simulink model "simscaptestworkspace"  (R2016b)
settings: Solver=VariableStepAuto  StartTime=0.0  StopTime=12100  RelTol=1e-3  AbsTol=1e-3  EnableMultiTasking=on
model workspace (MAT data in the model file):
  OCVdisch = [0  3.706; 5  3.337; 10  3.333; 15  3.331; 20  3.33; 25  3.329; 30  3.3284; 35  3.3272; 40  3.3237; 45  3.309; 50  3.2985; 55  3.295; 60  3.293; 65  3.2914; 70  3.2913; 75  3.2898; 80  3.2878; 85  3.2852; 90  3.2747; 95  3.259; 100  3.249; 105  3.2412; 110  3.231; 115  3.2172; 120  3.1983; 125  3.1673; 130  3.042; 132.5  2.9]
  Var = 1
undefined symbols (not defined in the file): C1, C2, C3, DOD, DOD1, OCV, R0, R1, R2, R3, sigbuilder_block
libraries: nesl_utility x11, fl_lib x8, elec_lib x3
settings Model: Creator=Karel Van Peteghem  LastModifiedBy=Karel Van Peteghem
settings DataIOCC: LimitDataPoints=on
settings OptimizationCC: LifeSpan=inf
settings DebuggingCC: AllowSymbolicDim=off  SFUnexpectedBacktrackingDiag=warning  SFNoUnconditionalDefaultTransitionDiag=warning  SFExecutionAtInitializationDiag=none
settings GRTTargetCC: TargetLangStandard=C89/C90 (ANSI)  GeneratePreprocessorConditionals=Disable all
settings ConfigComp: CovMetricSettings=dw  CovHtmlReporting=on  CovSaveCumulativeToWorkspaceVar=on  CovSaveSingleToWorkspaceVar=on  CovExternalEMLEnable=off  CovSFcnEnable=off
settings SimscapeCC: SimscapeLogType=all  SimscapeLogDataHistory=10000

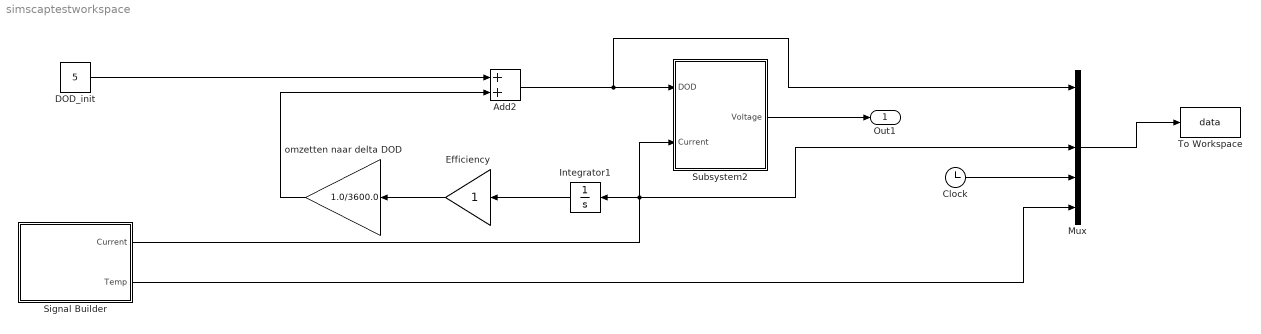
== system simscaptestworkspace ==
  Add2 : Sum
  Clock : Clock
  "DOD_init " : Constant  Value=5
  Efficiency : Gain
  Integrator1 : Integrator
  Mux : Mux  Inputs=5
  Signal Builder : Subsystem  Tag=STV Subsys  LoadFcn=sigbuilder_block('load');  StartFcn=sigbuilder_block('start');  StopFcn=sigbuilder_block('stop');  ClipboardFcn=sigbuilder_block('clipboard');  mask(Sigbuilder block){tuvar=[0:10]}
      mask help: Simulink:masks:SigbuilderBlock_MD
      mask init:
      | if ~strcmp(get_param(bdroot(gcbh),'SimulationStatus'),'stopped') tuvar = sigbuilder_block('maskInit'); end
      settings: CopyFcn=sigbuilder_block('copy');  DeleteFcn=sigbuilder_block('delete');  ModelCloseFcn=sigbuilder_block('modelClose');  PreSaveFcn=sigbuilder_block('preSave');  PauseFcn=sigbuilder_block('pause');  ContinueFcn=sigbuilder_block('continue');  NameChangeFcn=sigbuilder_block('namechange');  OpenFcn=sigbuilder_block('open',[228 111.75 550.5 359.25 ]);  CloseFcn=sigbuilder_block('close');
      mask Display: plot(0, 0, 100, 100,[2, 2, 32, 32, 2], [68, 8, 8, 68, 68],[32, 2], [38, 38], [32, 19, 2],[53, 60, 44], [32, 17, 17, 2],[16, 16, 31, 31]);txt = getActiveGroup(gcbh);text(2, 100, txt,'verticalAlignment', 'top');
  Subsystem2 : Subsystem
  To Workspace : ToWorkspace  VariableName=data  SampleTime=1
  omzetten naar delta DOD : Gain  Gain=1.0/3600.0
  Out1 : Outport
  wires:
  Mux/1 -> To Workspace/1
  "DOD_init "/1 -> Add2/1
  Add2/1 -> Mux/1, Subsystem2/1(DOD)
  Efficiency/1 -> omzetten naar delta DOD/1
  omzetten naar delta DOD/1 -> Add2/2
  Signal Builder/1(Current) -> Mux/3, Integrator1/1, Subsystem2/2(Current)
  Integrator1/1 -> Efficiency/1
  Clock/1 -> Mux/4
  Signal Builder/2(Temp) -> Mux/5
  Subsystem2/1(Voltage) -> Out1/1

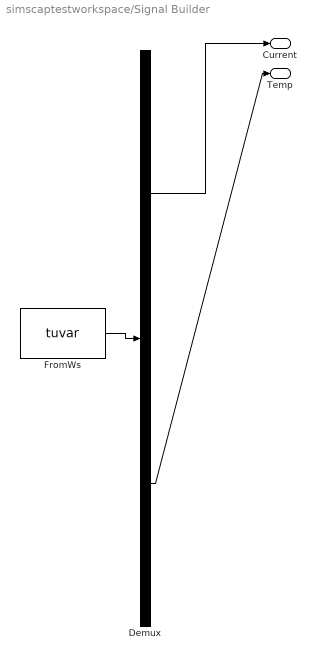
== system simscaptestworkspace/Signal Builder ==
  Demux : Demux  Tag=STV Demux  Outputs=2
  FromWs : FromWorkspace  Tag=STV FromWs  VariableName=tuvar  SampleTime=0
      SigBuilderData=|
      | common.afterFinalStr = 'Extrapolate'
      | common.sampleTime = 0
      | dataSet.timeRange = [0 12000]
      | dataSet.name = 'Blad1'
      | sbobj.Name = 'Signal Builder'
      | sbobj.Groups.Name = 'Blad1'
      | sbobj.Groups.Signals(1).Name = 'Current'
      | sbobj.Groups.Signals(1).XData = [0 101 101 1277 1277 12000]
      | sbobj.Groups.Signals(1).YData = [0 0 15 15 0 0]
      | sbobj.Groups.Signals(2).Name = 'Temp'
      | sbobj.Groups.Signals(2).XData = [0 101 101 1277 1277 12000]
      | sbobj.Groups.Signals(2).YData = [25 25 25 25 25 25]
      | sbobj.Groups.TimeRange = [0 12000]
  Current : Outport  Tag=STV Outport
  Temp : Outport  Tag=STV Outport  Port=2
  wires:
  Demux/1 -> Current/1
  FromWs/1 -> Demux/1
  Demux/2 -> Temp/1

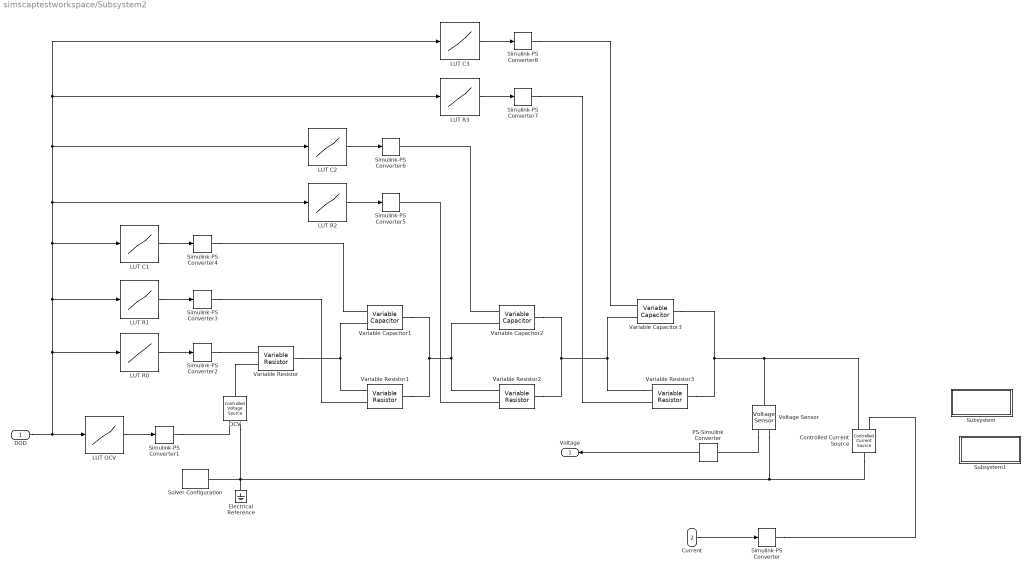
== system simscaptestworkspace/Subsystem2 ==
  DOD : Inport
  Current : Inport  Port=2
  Controlled Current Source : fl_lib/Electrical/Electrical Sources/Controlled Current Source
  Electrical Reference : fl_lib/Electrical/Electrical Elements/Electrical Reference
  LUT C1 : Lookup_n-D  NumberOfTableDimensions=1  LookupTableObject=OCVaangepast  BreakpointsForDimension1=DOD1  Table=C1  InternalRulePriority=Speed  RndMeth=Simplest  InputSameDT=on
  "LUT C2 " : Lookup_n-D  NumberOfTableDimensions=1  LookupTableObject=OCVaangepast  BreakpointsForDimension1=DOD1  Table=C2  InternalRulePriority=Speed  RndMeth=Simplest  InputSameDT=on
  LUT C3 : Lookup_n-D  NumberOfTableDimensions=1  LookupTableObject=OCVaangepast  BreakpointsForDimension1=DOD1  Table=C3  InternalRulePriority=Speed  RndMeth=Simplest  InputSameDT=on
  LUT OCV : Lookup_n-D  NumberOfTableDimensions=1  LookupTableObject=OCVaangepast  BreakpointsForDimension1=DOD  Table=OCV  InternalRulePriority=Speed  RndMeth=Simplest  InputSameDT=on
  LUT R0 : Lookup_n-D  NumberOfTableDimensions=1  LookupTableObject=OCVaangepast  BreakpointsForDimension1=DOD1  Table=R0  InternalRulePriority=Speed  RndMeth=Simplest  InputSameDT=on
  LUT R1 : Lookup_n-D  NumberOfTableDimensions=1  LookupTableObject=OCVaangepast  BreakpointsForDimension1=DOD1  Table=R1  InternalRulePriority=Speed  RndMeth=Simplest  InputSameDT=on
  LUT R2 : Lookup_n-D  NumberOfTableDimensions=1  LookupTableObject=OCVaangepast  BreakpointsForDimension1=DOD1  Table=R2  InternalRulePriority=Speed  RndMeth=Simplest  InputSameDT=on
  LUT R3 : Lookup_n-D  NumberOfTableDimensions=1  LookupTableObject=OCVaangepast  BreakpointsForDimension1=DOD1  Table=R3  InternalRulePriority=Speed  RndMeth=Simplest  InputSameDT=on
  OCV : fl_lib/Electrical/Electrical Sources/Controlled Voltage Source
  PS-Simulink Converter : nesl_utility/PS-Simulink Converter  PhysicalDomain=network_engine_domain  SubClassName=ps_output  LeftPortType=input  RightPortType=output  PseudoPeriodic=off  Frequencies=[]  Unit=1  AffineConversion=off
  Simulink-PS Converter{,1..8} (9 alike) : nesl_utility/Simulink-PS Converter  PhysicalDomain=network_engine_domain  SubClassName=ps_input  LeftPortType=input  RightPortType=output  PseudoPeriodic=off  Frequencies=[]  NoiseDistribution=none  NoiseParameters=[]  Unit=1  AffineConversion=off  InputFiltering=off  SimscapeFilterOrder=1  InputFilterTimeConstant=0.001  UdotUserProvided=1
  Solver Configuration : nesl_utility/Solver Configuration  PhysicalDomain=network_engine_domain  SubClassName=solver  LeftPortType=input  RightPortType=generic  Accelerate=off  Tones=[]  Harmonics=[]  SimulateNoise=off  Profile=off  UseLocalSampling=off  EnableSwitchedLinearOptims=on  FrequencyDomain=off  UseCCode=off  RelTol=0.001  AbsTol=1e-06  MinStep=1e-09  ToWorkspace=off  RevertToSquareIcSolve=off  NumHomotopyIterations=100  PhasorMode=off  PhasorModeNumHarmonics=1  OverrideAbsTol=off  DoDC=off  ResidualTolerance=1e-09  UseLocalSolver=off  LocalSolverChoice=NE_BACKWARD_EULER_ADVANCER  LocalSolverSampleTime=0.001  DoFixedCost=off  MaxNonlinIter=3  MaxModeIter=2  LinearAlgebra=Sparse  DelaysMemoryBudget=1024  AutomaticFiltering=on  FilteringTimeConstant=0.001
  Subsystem : Subsystem
      settings: OpenFcn=open_system('simscape')
      mask Display: disp(sprintf('Open Simscape\nLibrary'));
  Subsystem1 : Subsystem
      settings: OpenFcn=|
      | load_system('fl_lib');
      | open_system('fl_lib/Electrical');
      mask Display: disp(sprintf('Open Electrical\nLibrary'));
  Variable Capacitor1 : elec_lib/Passive Devices/Variable Capacitor  prm=2  Cmin=1e-9 F  r=0 Ohm  v0=0 V  q0=0 C
  Variable Capacitor2 : elec_lib/Passive Devices/Variable Capacitor  prm=2  Cmin=1e-9 F  r=0 Ohm  v0=0 V  q0=0 C
  Variable Capacitor3 : elec_lib/Passive Devices/Variable Capacitor  prm=2  Cmin=1e-9 F  r=0 Ohm  v0=0 V  q0=0 C
  Variable Resistor{,1..3} (4 alike) : fl_lib/Electrical/Electrical Elements/Variable Resistor  Rmin=0 Ohm  i_specify=off  i_priority=None  i=0 A  v_specify=off  v_priority=None  v=0 V
  Voltage Sensor : fl_lib/Electrical/Electrical Sensors/Voltage Sensor
  Voltage : Outport
  wires:
  Current/1 -> Simulink-PS Converter/1
  PS-Simulink Converter/1 -> Voltage/1
  LUT OCV/1 -> Simulink-PS Converter1/1
  LUT R0/1 -> Simulink-PS Converter2/1
  LUT R1/1 -> Simulink-PS Converter3/1
  LUT C1/1 -> Simulink-PS Converter4/1
  LUT R2/1 -> Simulink-PS Converter5/1
  "LUT C2 "/1 -> Simulink-PS Converter6/1
  DOD/1 -> LUT OCV/1, LUT R1/1, LUT C3/1, LUT R3/1, "LUT C2 "/1, LUT R2/1, LUT C1/1, LUT R0/1
  LUT R3/1 -> Simulink-PS Converter7/1
  LUT C3/1 -> Simulink-PS Converter8/1
  connections:
  Variable Resistor/RConn1 -- Variable Resistor1/LConn2 -- Variable Capacitor1/LConn2
  Electrical Reference/LConn1 -- Voltage Sensor/RConn2 -- Controlled Current Source/LConn1 -- OCV/RConn2 -- Solver Configuration/RConn1
  Variable Capacitor1/RConn1 -- Variable Capacitor2/LConn2 -- Variable Resistor2/LConn2 -- Variable Resistor1/RConn1
  Simulink-PS Converter1/RConn1 -- OCV/RConn1
  Variable Resistor/LConn2 -- OCV/LConn1
  Simulink-PS Converter/RConn1 -- Controlled Current Source/RConn1
  Variable Capacitor3/RConn1 -- Variable Resistor3/RConn1 -- Controlled Current Source/RConn2 -- Voltage Sensor/LConn1
  Voltage Sensor/RConn1 -- PS-Simulink Converter/LConn1
  Simulink-PS Converter2/RConn1 -- Variable Resistor/LConn1
  Simulink-PS Converter3/RConn1 -- Variable Resistor1/LConn1
  Simulink-PS Converter4/RConn1 -- Variable Capacitor1/LConn1
  Variable Resistor3/LConn2 -- Variable Capacitor3/LConn2 -- Variable Resistor2/RConn1 -- Variable Capacitor2/RConn1
  Variable Resistor2/LConn1 -- Simulink-PS Converter5/RConn1
  Variable Capacitor2/LConn1 -- Simulink-PS Converter6/RConn1
  Simulink-PS Converter8/RConn1 -- Variable Capacitor3/LConn1
  Simulink-PS Converter7/RConn1 -- Variable Resistor3/LConn1

== system simscaptestworkspace/Subsystem2/Subsystem ==

== system simscaptestworkspace/Subsystem2/Subsystem1 ==
